simulink model "PID_Simulink_2DOF"  (R2019a)
settings: Solver=VariableStepAuto  StartTime=0.0  StopTime=250  RelTol=1e-3
undefined symbols (not defined in the file): A, A_d, B, B_d, C, C_d, DiscIntNeverNeededParam, Ki, Ki_d, Kx, Kx_d, Ts
libraries: simulink x6
settings Model: Creator=Caeta  LastModifiedBy=Caeta

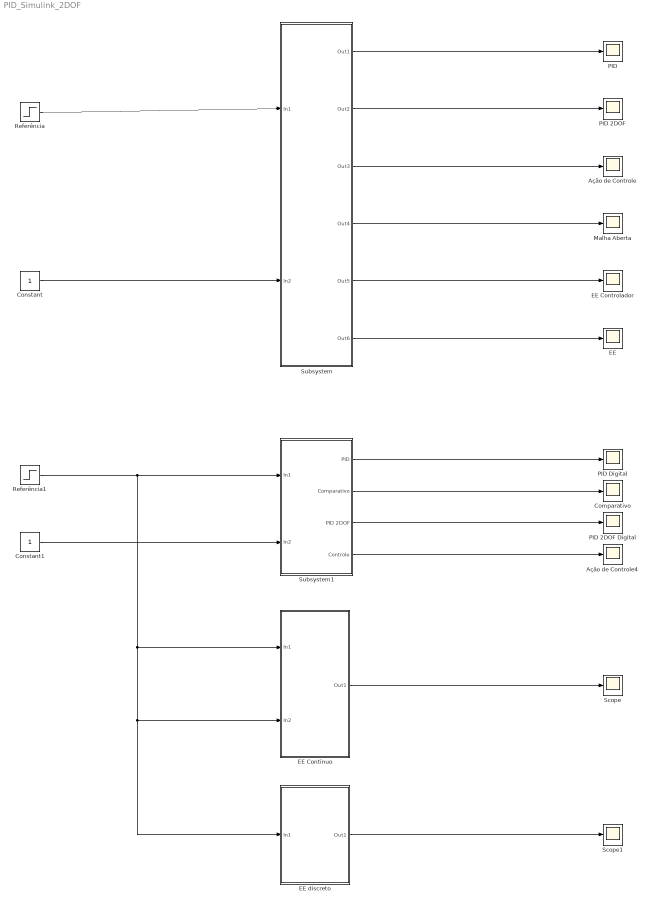
== system PID_Simulink_2DOF ==
  Ação de Controle : Scope
  Ação de Controle4 : Scope
  Comparativo : Scope
  Constant : Constant
  Constant1 : Constant
  "EE " : Scope
  EE Controlador : Scope
  EE Contínuo : Subsystem
  EE discreto : Subsystem
  Malha Aberta : Scope
  PID : Scope
  PID 2DOF : Scope
  PID 2DOF Digital : Scope
  PID Digital : Scope
  Referência : Step  Time=0  SampleTime=0
  Referência1 : Step  Time=0  SampleTime=Ts
  Scope : Scope
  Scope1 : Scope
  Subsystem : Subsystem
  Subsystem1 : Subsystem
  wires:
  Referência/1 -> Subsystem/1(In1)
  Constant/1 -> Subsystem/2(In2)
  Subsystem/1(Out1) -> PID/1
  Subsystem/2(Out2) -> PID 2DOF/1
  Subsystem/3(Out3) -> Ação de Controle/1
  Subsystem/4(Out4) -> Malha Aberta/1
  Subsystem/5(Out5) -> EE Controlador/1
  Subsystem/6(Out6) -> "EE "/1
  Constant1/1 -> Subsystem1/2(In2)
  Subsystem1/1(PID) -> PID Digital/1
  Subsystem1/2(Comparativo) -> Comparativo/1
  Subsystem1/3(PID 2DOF) -> PID 2DOF Digital/1
  Subsystem1/4(Controle) -> Ação de Controle4/1
  Referência1/1 -> EE Contínuo/1(In1), EE discreto/1(In1), EE Contínuo/2(In2), Subsystem1/1(In1)
  EE Contínuo/1(Out1) -> Scope/1
  EE discreto/1(Out1) -> Scope1/1

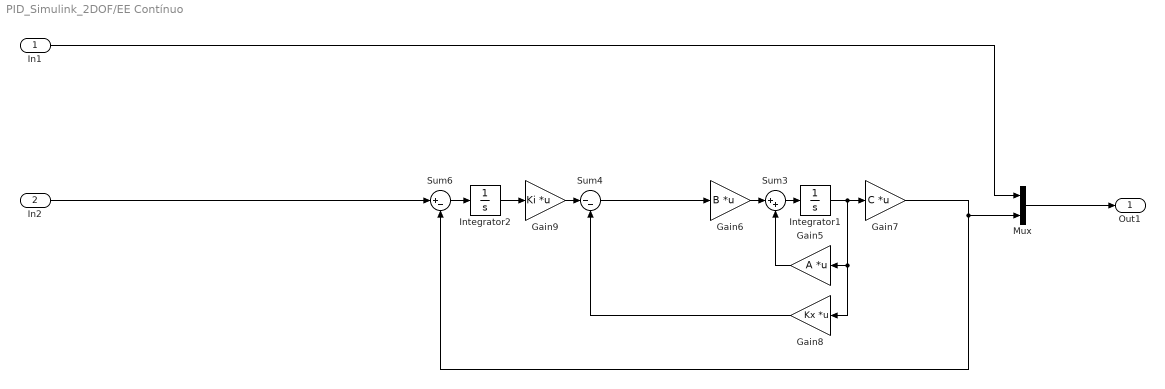
== system PID_Simulink_2DOF/EE Contínuo ==
  In1 : Inport
  In2 : Inport  Port=2
  Gain5 : Gain  Gain=A  Multiplication=Matrix(K*u)
  Gain6 : Gain  Gain=B  Multiplication=Matrix(K*u)
  Gain7 : Gain  Gain=C  Multiplication=Matrix(K*u)
  Gain8 : Gain  Gain=Kx  Multiplication=Matrix(K*u)
  Gain9 : Gain  Gain=Ki  Multiplication=Matrix(K*u)
  Integrator1 : Integrator
  Integrator2 : Integrator
  Mux : Mux  Inputs=2
  Sum3 : Sum  Inputs=|++
  Sum4 : Sum  Inputs=|--
  Sum6 : Sum  Inputs=|+-
  Out1 : Outport
  wires:
  Gain7/1 -> Mux/2, Sum6/2
  Gain9/1 -> Sum4/1
  Sum6/1 -> Integrator2/1
  Gain8/1 -> Sum4/2
  Integrator1/1 -> Gain8/1, Gain5/1, Gain7/1
  Gain6/1 -> Sum3/1
  Gain5/1 -> Sum3/2
  Sum3/1 -> Integrator1/1
  Integrator2/1 -> Gain9/1
  Sum4/1 -> Gain6/1
  In2/1 -> Sum6/1
  In1/1 -> Mux/1
  Mux/1 -> Out1/1

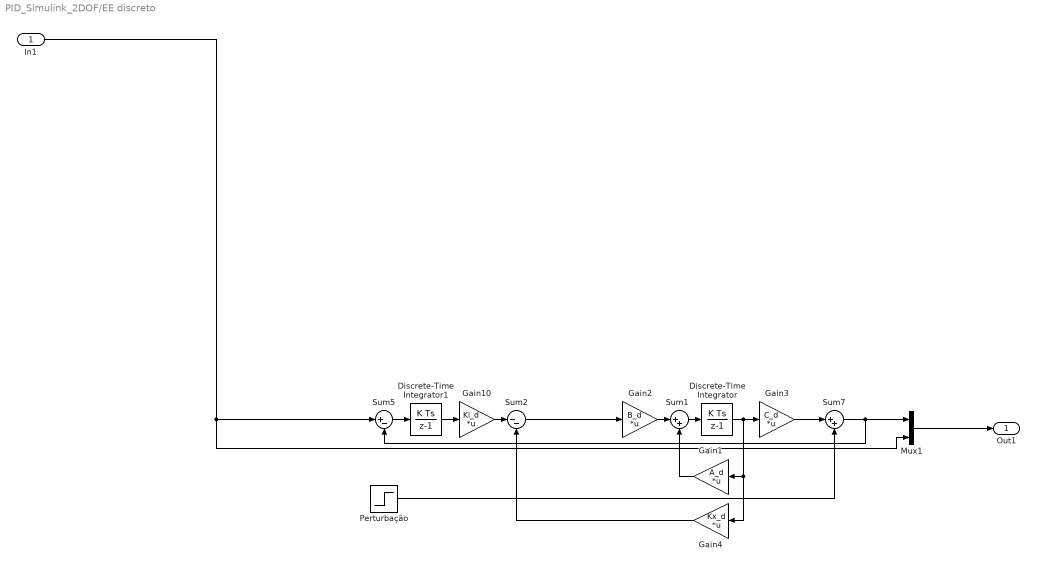
== system PID_Simulink_2DOF/EE discreto ==
  In1 : Inport
  Discrete-Time Integrator : DiscreteIntegrator  SampleTime=Ts  ICPrevOutput=DiscIntNeverNeededParam  ICPrevScaledInput=DiscIntNeverNeededParam
  Discrete-Time Integrator1 : DiscreteIntegrator  SampleTime=Ts  ICPrevOutput=DiscIntNeverNeededParam  ICPrevScaledInput=DiscIntNeverNeededParam
  Gain1 : Gain  Gain=A_d  Multiplication=Matrix(K*u)
  Gain10 : Gain  Gain=Ki_d  Multiplication=Matrix(K*u)
  Gain2 : Gain  Gain=B_d  Multiplication=Matrix(K*u)
  Gain3 : Gain  Gain=C_d  Multiplication=Matrix(K*u)
  Gain4 : Gain  Gain=Kx_d  Multiplication=Matrix(K*u)
  Mux1 : Mux  Inputs=2
  Perturbação : Step  Time=150  After=0.1  SampleTime=Ts
  Sum1 : Sum  Inputs=|++
  Sum2 : Sum  Inputs=|--
  Sum5 : Sum  Inputs=|+-
  Sum7 : Sum  Inputs=|++
  Out1 : Outport
  wires:
  Sum7/1 -> Mux1/1, Sum5/2
  Perturbação/1 -> Sum7/2
  Gain2/1 -> Sum1/1
  Gain10/1 -> Sum2/1
  Discrete-Time Integrator/1 -> Gain4/1, Gain1/1, Gain3/1
  Discrete-Time Integrator1/1 -> Gain10/1
  Mux1/1 -> Out1/1
  Gain4/1 -> Sum2/2
  Sum1/1 -> Discrete-Time Integrator/1
  In1/1 -> Mux1/2, Sum5/1
  Sum5/1 -> Discrete-Time Integrator1/1
  Gain1/1 -> Sum1/2
  Sum2/1 -> Gain2/1
  Gain3/1 -> Sum7/1

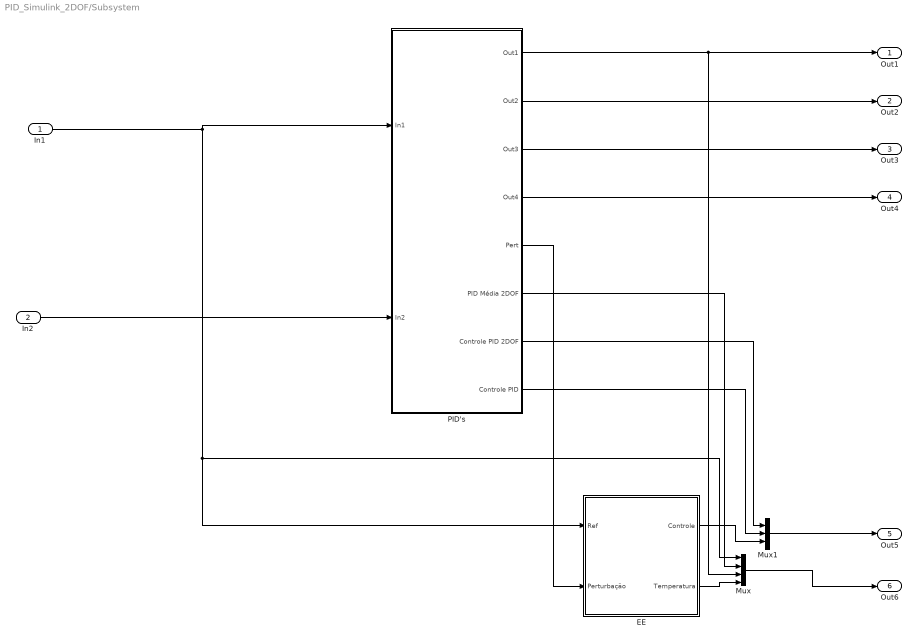
== system PID_Simulink_2DOF/Subsystem ==
  In1 : Inport
  In2 : Inport  Port=2
  EE : Subsystem
  Mux : Mux
  Mux1 : Mux  Inputs=3
  PID's : Subsystem
  Out1 : Outport
  Out2 : Outport  Port=2
  Out3 : Outport  Port=3
  Out4 : Outport  Port=4
  Out5 : Outport  Port=5
  Out6 : Outport  Port=6
  wires:
  PID's/3(Out3) -> Out3/1
  PID's/8(Controle PID) -> Mux1/2
  Mux1/1 -> Out5/1
  PID's/6(PID Média 2DOF) -> Mux/2
  In1/1 -> Mux/1, EE/1(Ref), PID's/1(In1)
  PID's/5(Pert) -> EE/2(Perturbação)
  PID's/7(Controle PID 2DOF) -> Mux1/1
  PID's/1(Out1) -> Out1/1, Mux/3
  PID's/4(Out4) -> Out4/1
  PID's/2(Out2) -> Out2/1
  In2/1 -> PID's/2(In2)
  Mux/1 -> Out6/1
  EE/1(Controle) -> Mux1/3
  EE/2(Temperatura) -> Mux/4

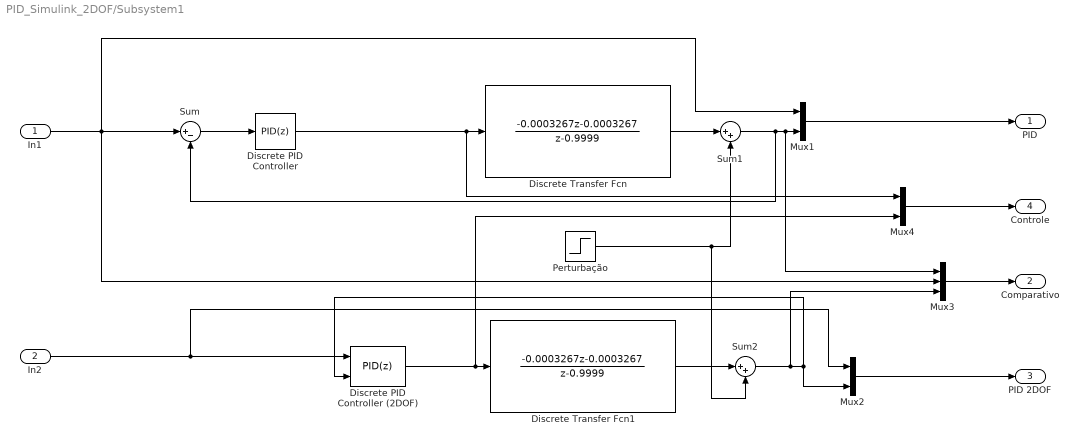
== system PID_Simulink_2DOF/Subsystem1 ==
  In1 : Inport
  In2 : Inport  Port=2
  Discrete Transfer Fcn : DiscreteTransferFcn  Numerator=[-0.0003267 -0.0003267]  Denominator=[1 -0.9999]  SampleTime=Ts
  Discrete Transfer Fcn1 : DiscreteTransferFcn  Numerator=[-0.0003267 -0.0003267]  Denominator=[1 -0.9999]  SampleTime=Ts
  Discrete PID Controller : simulink/Continuous/PID Controller  Controller=PID  Form=Parallel  TimeDomain=Discrete-time  SampleTime=Ts  IntegratorMethod=Forward Euler  FilterMethod=Forward Euler  ControllerParametersSource=internal  P=-38  I=-3  D=-0.1  UseFilter=off  N=0  TunerSelectOption=Transfer Function Based (PID Tuner App)  InitialConditionSource=internal  InitialConditionForIntegrator=0  InitialConditionForFilter=0  DifferentiatorICPrevScaledInput=0  ExternalReset=none  TrackingMode=off  Kt=1  LimitOutput=off  UpperSaturationLimit=inf  LowerSaturationLimit=-inf  LinearizeAsGain=off  AntiWindupMode=none  Kb=1  POutMin=[]  POutMax=[]  IOutMin=[]  IOutMax=[]  DOutMin=[]  DOutMax=[]  NOutMin=[]  NOutMax=[]  SumOutMin=[]  SumOutMax=[]  SaturationOutMin=[]  SaturationOutMax=[]  PParamMin=[]  PParamMax=[]  IParamMin=[]  IParamMax=[]  DParamMin=[]  DParamMax=[]  NParamMin=[]  NParamMax=[]  KbParamMin=[]  KbParamMax=[]  KtParamMin=[]  KtParamMax=[]  KbOutMin=[]  KbOutMax=[]  KtOutMin=[]  KtOutMax=[]  IntegratorOutMin=[]  IntegratorOutMax=[]  FilterOutMin=[]  FilterOutMax=[]  SumI1OutMin=[]  SumI1OutMax=[]  SumI2OutMin=[]  SumI2OutMax=[]  SumI3OutMin=[]  SumI3OutMax=[]  SumI4OutMin=[]  SumI4OutMax=[]  SumDOutMin=[]  SumDOutMax=[]  DifferentiatorOutMin=[]  DifferentiatorOutMax=[]  FilterDiffOutCoefMin=[]  FilterDiffOutCoefMax=[]  ReciprocalOutMin=[]  ReciprocalOutMax=[]  SumDenOutMin=[]  SumDenOutMax=[]  SumNumOutMin=[]  SumNumOutMax=[]  DivideOutMin=[]  DivideOutMax=[]  IntegratorContinuousStateAttributes=''  IntegratorStateMustResolveToSignalObject=off  IntegratorRTWStateStorageClass=Auto  FilterContinuousStateAttributes=''  FilterStateMustResolveToSignalObject=off  FilterRTWStateStorageClass=Auto  ParallelPVariant=InternalParameters  IdealPVariant=Disabled  IVariant=InternalParameters  DVariant=InternalParameters  IntegratorVariant=Discrete  SatVariant=Disabled  AWVariant=Passthrough  PCopyVariant=Disabled  TRVariant=Disabled  FdbkBlocksVariant=Forward  IdealPFdbkVariant=Disabled  SatFdbkVariant=Disabled  DerivativeFilterVariant=Differentiator  NVariant=Passthrough  NCopyVariant=Disabled_SignalSpec  FilterICVariant=InternalICsDifferentiator  IntegratorICVariant=InternalICs  ExternalResetVariant=Disabled  TRSumVariant=Passthrough  SumFdbkVariant=Disabled  SumVariant=Sum_PID
  Discrete PID Controller (2DOF) : simulink/Continuous/PID Controller (2DOF)  Controller=PID  Form=Parallel  TimeDomain=Discrete-time  SampleTime=Ts  IntegratorMethod=Forward Euler  FilterMethod=Forward Euler  ControllerParametersSource=internal  P=-38  I=-3  D=-0.1  UseFilter=on  N=0  b=0.8  c=0.8  TunerSelectOption=Transfer Function Based (PID Tuner App)  InitialConditionSource=internal  InitialConditionForIntegrator=0  InitialConditionForFilter=0  DifferentiatorICPrevScaledInput=0  ExternalReset=none  TrackingMode=off  Kt=1  LimitOutput=off  UpperSaturationLimit=inf  LowerSaturationLimit=-inf  LinearizeAsGain=off  AntiWindupMode=none  Kb=1  POutMin=[]  POutMax=[]  IOutMin=[]  IOutMax=[]  DOutMin=[]  DOutMax=[]  NOutMin=[]  NOutMax=[]  bOutMin=[]  bOutMax=[]  cOutMin=[]  cOutMax=[]  SumOutMin=[]  SumOutMax=[]  SaturationOutMin=[]  SaturationOutMax=[]  PParamMin=[]  PParamMax=[]  IParamMin=[]  IParamMax=[]  DParamMin=[]  DParamMax=[]  NParamMin=[]  NParamMax=[]  bParamMin=[]  bParamMax=[]  cParamMin=[]  cParamMax=[]  KbParamMin=[]  KbParamMax=[]  KtParamMin=[]  KtParamMax=[]  KbOutMin=[]  KbOutMax=[]  KtOutMin=[]  KtOutMax=[]  IntegratorOutMin=[]  IntegratorOutMax=[]  FilterOutMin=[]  FilterOutMax=[]  SumI1OutMin=[]  SumI1OutMax=[]  SumI2OutMin=[]  SumI2OutMax=[]  SumI3OutMin=[]  SumI3OutMax=[]  SumI4OutMin=[]  SumI4OutMax=[]  SumDOutMin=[]  SumDOutMax=[]  Sum1OutMin=[]  Sum1OutMax=[]  Sum2OutMin=[]  Sum2OutMax=[]  Sum3OutMin=[]  Sum3OutMax=[]  DifferentiatorOutMin=[]  DifferentiatorOutMax=[]  FilterDiffOutCoefMin=[]  FilterDiffOutCoefMax=[]  ReciprocalOutMin=[]  ReciprocalOutMax=[]  SumDenOutMin=[]  SumDenOutMax=[]  SumNumOutMin=[]  SumNumOutMax=[]  DivideOutMin=[]  DivideOutMax=[]  IntegratorContinuousStateAttributes=''  IntegratorStateMustResolveToSignalObject=off  IntegratorRTWStateStorageClass=Auto  FilterContinuousStateAttributes=''  FilterStateMustResolveToSignalObject=off  FilterRTWStateStorageClass=Auto  ParallelPVariant=InternalParameters  IdealPVariant=Disabled  IVariant=InternalParameters  DVariant=InternalParameters  bVariant=InternalParameters  cVariant=InternalParameters  IntegratorVariant=Discrete  SatVariant=Disabled  AWVariant=Passthrough  PCopyVariant=Disabled  TRVariant=Disabled  FdbkBlocksVariant=Forward  IdealPFdbkVariant=Disabled  SatFdbkVariant=Disabled  DerivativeFilterVariant=ForwardEulerFilter  NVariant=InternalParameters  NCopyVariant=Disabled  FilterICVariant=InternalICsFilter  IntegratorICVariant=InternalICs  ExternalResetVariant=Disabled  TRSumVariant=Passthrough  SumFdbkVariant=Disabled  SumVariant=Sum_PID
  Mux1 : Mux  Inputs=2
  Mux2 : Mux  Inputs=2
  Mux3 : Mux  Inputs=3
  Mux4 : Mux  Inputs=2
  Perturbação : Step  Time=50  After=0.1  SampleTime=Ts
  Sum : Sum  Inputs=|+-
  Sum1 : Sum  Inputs=|++
  Sum2 : Sum  Inputs=|++
  PID : Outport
  Comparativo : Outport  Port=2
  PID 2DOF : Outport  Port=3
  Controle : Outport  Port=4
  wires:
  Sum2/1 -> Mux3/3, Mux2/2, Discrete PID Controller (2DOF)/2
  Discrete Transfer Fcn/1 -> Sum1/1
  In1/1 -> Mux3/2, Mux1/1, Sum/1
  Sum/1 -> Discrete PID Controller/1
  In2/1 -> Mux2/1, Discrete PID Controller (2DOF)/1
  Perturbação/1 -> Sum2/2, Sum1/2
  Sum1/1 -> Sum/2, Mux3/1, Mux1/2
  Discrete Transfer Fcn1/1 -> Sum2/1
  Mux3/1 -> Comparativo/1
  Mux1/1 -> PID/1
  Mux2/1 -> PID 2DOF/1
  Discrete PID Controller (2DOF)/1 -> Mux4/2, Discrete Transfer Fcn1/1
  Discrete PID Controller/1 -> Mux4/1, Discrete Transfer Fcn/1
  Mux4/1 -> Controle/1

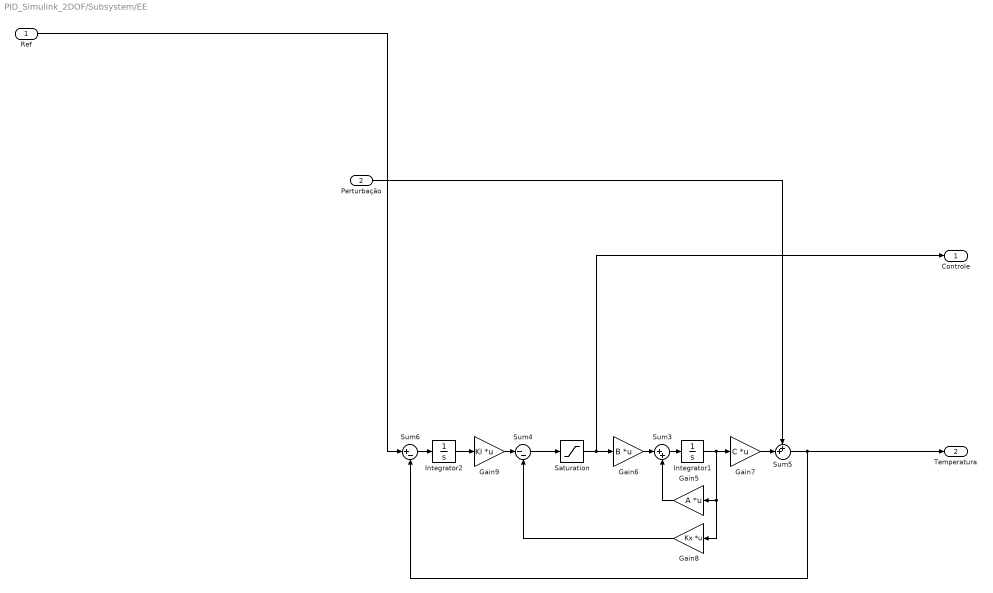
== system PID_Simulink_2DOF/Subsystem/EE ==
  Ref : Inport
  Perturbação : Inport  Port=2
  Gain5 : Gain  Gain=A  Multiplication=Matrix(K*u)
  Gain6 : Gain  Gain=B  Multiplication=Matrix(K*u)
  Gain7 : Gain  Gain=C  Multiplication=Matrix(K*u)
  Gain8 : Gain  Gain=Kx  Multiplication=Matrix(K*u)
  Gain9 : Gain  Gain=Ki  Multiplication=Matrix(K*u)
  Integrator1 : Integrator
  Integrator2 : Integrator
  Saturation : Saturate  UpperLimit=255  LowerLimit=0
  Sum3 : Sum  Inputs=|++
  Sum4 : Sum  Inputs=|--
  Sum5 : Sum  Inputs=++|
  Sum6 : Sum  Inputs=|+-
  Controle : Outport
  Temperatura : Outport  Port=2
  wires:
  Sum3/1 -> Integrator1/1
  Sum5/1 -> Sum6/2, Temperatura/1
  Gain9/1 -> Sum4/1
  Integrator2/1 -> Gain9/1
  Sum6/1 -> Integrator2/1
  Gain6/1 -> Sum3/1
  Gain7/1 -> Sum5/2
  Gain8/1 -> Sum4/2
  Integrator1/1 -> Gain8/1, Gain5/1, Gain7/1
  Gain5/1 -> Sum3/2
  Perturbação/1 -> Sum5/1
  Ref/1 -> Sum6/1
  Sum4/1 -> Saturation/1
  Saturation/1 -> Controle/1, Gain6/1

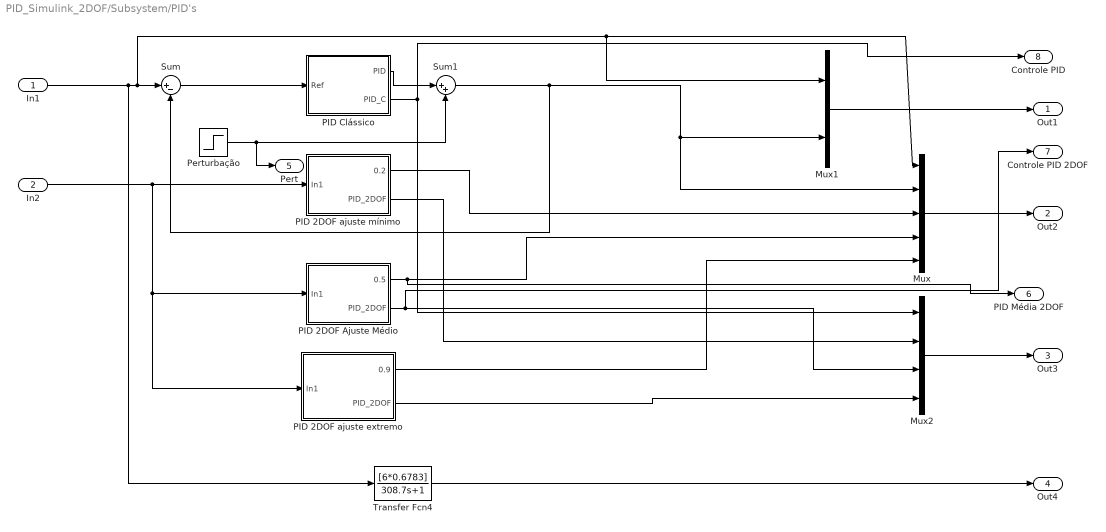
== system PID_Simulink_2DOF/Subsystem/PID's ==
  In1 : Inport
  In2 : Inport  Port=2
  Mux : Mux  Inputs=5
  Mux1 : Mux  Inputs=2
  Mux2 : Mux
  PID 2DOF Ajuste Médio : Subsystem
  PID 2DOF ajuste extremo : Subsystem
  PID 2DOF ajuste mínimo : Subsystem
  PID Clássico : Subsystem
  Perturbação : Step  Time=150  After=0.1  SampleTime=0
  Sum : Sum  Inputs=|+-
  Sum1 : Sum  Inputs=|++
  Transfer Fcn4 : TransferFcn  Numerator=[6*0.6783]  Denominator=[308.7 1]
  Out1 : Outport
  Out2 : Outport  Port=2
  Out3 : Outport  Port=3
  Out4 : Outport  Port=4
  Pert : Outport  Port=5
  PID Média 2DOF : Outport  Port=6
  Controle PID 2DOF : Outport  Port=7
  Controle PID : Outport  Port=8
  wires:
  Sum/1 -> PID Clássico/1(Ref)
  In2/1 -> PID 2DOF Ajuste Médio/1(In1), PID 2DOF ajuste extremo/1(In1), PID 2DOF ajuste mínimo/1(In1)
  Sum1/1 -> Mux1/2, Mux/2, Sum/2
  Mux/1 -> Out2/1
  PID 2DOF Ajuste Médio/2(PID_2DOF) -> Controle PID 2DOF/1, Mux2/3
  In1/1 -> Transfer Fcn4/1, Mux1/1, Mux/1, Sum/1
  PID 2DOF ajuste mínimo/1(0.2) -> Mux/3
  Transfer Fcn4/1 -> Out4/1
  PID Clássico/1(PID) -> Sum1/1
  PID 2DOF Ajuste Médio/1(0.5) -> PID Média 2DOF/1, Mux/4
  PID 2DOF ajuste mínimo/2("PID_2DOF ") -> Mux2/2
  PID 2DOF ajuste extremo/2(PID_2DOF) -> Mux2/4
  PID Clássico/2(PID_C) -> Mux2/1, Controle PID/1
  PID 2DOF ajuste extremo/1("0.9 ") -> Mux/5
  Perturbação/1 -> Pert/1, Sum1/2
  Mux1/1 -> Out1/1
  Mux2/1 -> Out3/1

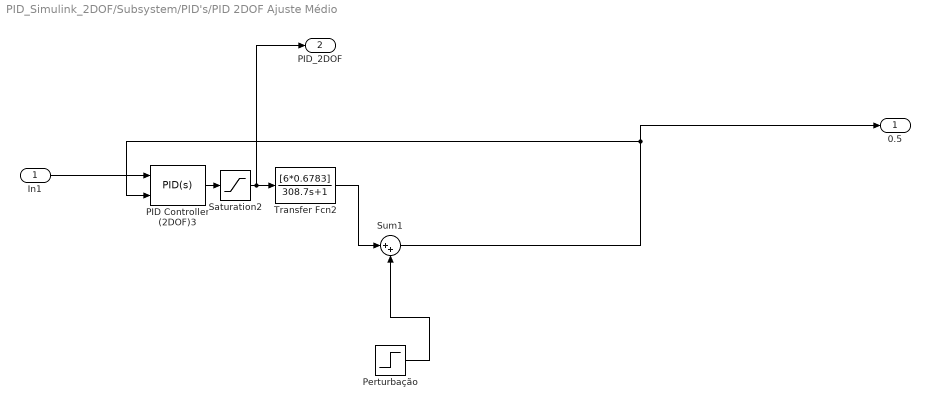
== system PID_Simulink_2DOF/Subsystem/PID's/PID 2DOF Ajuste Médio ==
  In1 : Inport
  PID Controller (2DOF)3 : simulink/Continuous/PID Controller (2DOF)  Controller=PID  Form=Parallel  TimeDomain=Continuous-time  SampleTime=-1  IntegratorMethod=Forward Euler  FilterMethod=Forward Euler  ControllerParametersSource=internal  P=7.03  I=0.182  D=25.1  UseFilter=on  N=0  b=0.5  c=0.5  TunerSelectOption=Transfer Function Based (PID Tuner App)  InitialConditionSource=internal  InitialConditionForIntegrator=0  InitialConditionForFilter=0  DifferentiatorICPrevScaledInput=0  ExternalReset=none  TrackingMode=off  Kt=1  LimitOutput=off  UpperSaturationLimit=inf  LowerSaturationLimit=-inf  LinearizeAsGain=on  AntiWindupMode=none  Kb=1  POutMin=[]  POutMax=[]  IOutMin=[]  IOutMax=[]  DOutMin=[]  DOutMax=[]  NOutMin=[]  NOutMax=[]  bOutMin=[]  bOutMax=[]  cOutMin=[]  cOutMax=[]  SumOutMin=[]  SumOutMax=[]  SaturationOutMin=[]  SaturationOutMax=[]  PParamMin=[]  PParamMax=[]  IParamMin=[]  IParamMax=[]  DParamMin=[]  DParamMax=[]  NParamMin=[]  NParamMax=[]  bParamMin=[]  bParamMax=[]  cParamMin=[]  cParamMax=[]  KbParamMin=[]  KbParamMax=[]  KtParamMin=[]  KtParamMax=[]  KbOutMin=[]  KbOutMax=[]  KtOutMin=[]  KtOutMax=[]  IntegratorOutMin=[]  IntegratorOutMax=[]  FilterOutMin=[]  FilterOutMax=[]  SumI1OutMin=[]  SumI1OutMax=[]  SumI2OutMin=[]  SumI2OutMax=[]  SumI3OutMin=[]  SumI3OutMax=[]  SumI4OutMin=[]  SumI4OutMax=[]  SumDOutMin=[]  SumDOutMax=[]  Sum1OutMin=[]  Sum1OutMax=[]  Sum2OutMin=[]  Sum2OutMax=[]  Sum3OutMin=[]  Sum3OutMax=[]  DifferentiatorOutMin=[]  DifferentiatorOutMax=[]  FilterDiffOutCoefMin=[]  FilterDiffOutCoefMax=[]  ReciprocalOutMin=[]  ReciprocalOutMax=[]  SumDenOutMin=[]  SumDenOutMax=[]  SumNumOutMin=[]  SumNumOutMax=[]  DivideOutMin=[]  DivideOutMax=[]  IntegratorContinuousStateAttributes=''  IntegratorStateMustResolveToSignalObject=off  IntegratorRTWStateStorageClass=Auto  FilterContinuousStateAttributes=''  FilterStateMustResolveToSignalObject=off  FilterRTWStateStorageClass=Auto  ParallelPVariant=InternalParameters  IdealPVariant=Disabled  IVariant=InternalParameters  DVariant=InternalParameters  bVariant=InternalParameters  cVariant=InternalParameters  IntegratorVariant=Continuous  SatVariant=Disabled  AWVariant=Passthrough  PCopyVariant=Disabled  TRVariant=Disabled  FdbkBlocksVariant=Forward  IdealPFdbkVariant=Disabled  SatFdbkVariant=Disabled  DerivativeFilterVariant=ContFilter  NVariant=InternalParameters  NCopyVariant=Disabled  FilterICVariant=InternalICsFilter  IntegratorICVariant=InternalICs  ExternalResetVariant=Disabled  TRSumVariant=Passthrough  SumFdbkVariant=Disabled  SumVariant=Sum_PID
  Perturbação : Step  Time=150  After=0.1  SampleTime=0
  Saturation2 : Saturate  UpperLimit=255  LowerLimit=0
  Sum1 : Sum  Inputs=|++
  Transfer Fcn2 : TransferFcn  Numerator=[6*0.6783]  Denominator=[308.7 1]
  0.5 : Outport
  PID_2DOF : Outport  Port=2
  wires:
  PID Controller (2DOF)3/1 -> Saturation2/1
  In1/1 -> PID Controller (2DOF)3/1
  Saturation2/1 -> PID_2DOF/1, Transfer Fcn2/1
  Perturbação/1 -> Sum1/2
  Transfer Fcn2/1 -> Sum1/1
  Sum1/1 -> 0.5/1, PID Controller (2DOF)3/2

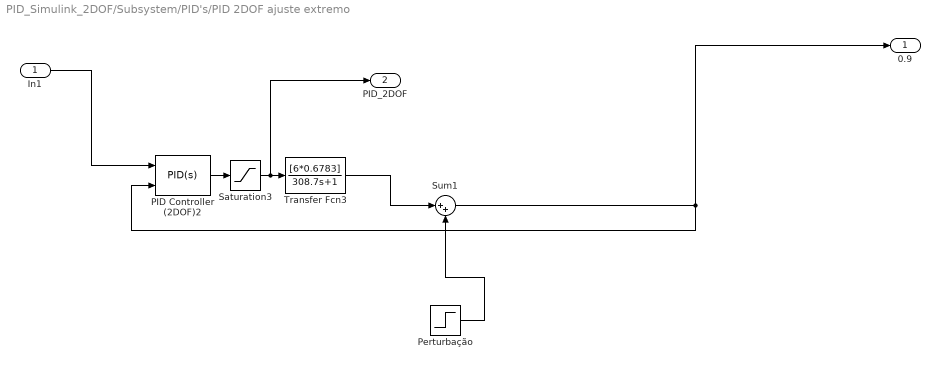
== system PID_Simulink_2DOF/Subsystem/PID's/PID 2DOF ajuste extremo ==
  In1 : Inport
  PID Controller (2DOF)2 : simulink/Continuous/PID Controller (2DOF)  Controller=PID  Form=Parallel  TimeDomain=Continuous-time  SampleTime=-1  IntegratorMethod=Forward Euler  FilterMethod=Forward Euler  ControllerParametersSource=internal  P=7.03  I=0.182  D=25.1  UseFilter=on  N=0  b=0.9  c=0.9  TunerSelectOption=Transfer Function Based (PID Tuner App)  InitialConditionSource=internal  InitialConditionForIntegrator=0  InitialConditionForFilter=0  DifferentiatorICPrevScaledInput=0  ExternalReset=none  TrackingMode=off  Kt=1  LimitOutput=off  UpperSaturationLimit=inf  LowerSaturationLimit=-inf  LinearizeAsGain=on  AntiWindupMode=none  Kb=1  POutMin=[]  POutMax=[]  IOutMin=[]  IOutMax=[]  DOutMin=[]  DOutMax=[]  NOutMin=[]  NOutMax=[]  bOutMin=[]  bOutMax=[]  cOutMin=[]  cOutMax=[]  SumOutMin=[]  SumOutMax=[]  SaturationOutMin=[]  SaturationOutMax=[]  PParamMin=[]  PParamMax=[]  IParamMin=[]  IParamMax=[]  DParamMin=[]  DParamMax=[]  NParamMin=[]  NParamMax=[]  bParamMin=[]  bParamMax=[]  cParamMin=[]  cParamMax=[]  KbParamMin=[]  KbParamMax=[]  KtParamMin=[]  KtParamMax=[]  KbOutMin=[]  KbOutMax=[]  KtOutMin=[]  KtOutMax=[]  IntegratorOutMin=[]  IntegratorOutMax=[]  FilterOutMin=[]  FilterOutMax=[]  SumI1OutMin=[]  SumI1OutMax=[]  SumI2OutMin=[]  SumI2OutMax=[]  SumI3OutMin=[]  SumI3OutMax=[]  SumI4OutMin=[]  SumI4OutMax=[]  SumDOutMin=[]  SumDOutMax=[]  Sum1OutMin=[]  Sum1OutMax=[]  Sum2OutMin=[]  Sum2OutMax=[]  Sum3OutMin=[]  Sum3OutMax=[]  DifferentiatorOutMin=[]  DifferentiatorOutMax=[]  FilterDiffOutCoefMin=[]  FilterDiffOutCoefMax=[]  ReciprocalOutMin=[]  ReciprocalOutMax=[]  SumDenOutMin=[]  SumDenOutMax=[]  SumNumOutMin=[]  SumNumOutMax=[]  DivideOutMin=[]  DivideOutMax=[]  IntegratorContinuousStateAttributes=''  IntegratorStateMustResolveToSignalObject=off  IntegratorRTWStateStorageClass=Auto  FilterContinuousStateAttributes=''  FilterStateMustResolveToSignalObject=off  FilterRTWStateStorageClass=Auto  ParallelPVariant=InternalParameters  IdealPVariant=Disabled  IVariant=InternalParameters  DVariant=InternalParameters  bVariant=InternalParameters  cVariant=InternalParameters  IntegratorVariant=Continuous  SatVariant=Disabled  AWVariant=Passthrough  PCopyVariant=Disabled  TRVariant=Disabled  FdbkBlocksVariant=Forward  IdealPFdbkVariant=Disabled  SatFdbkVariant=Disabled  DerivativeFilterVariant=ContFilter  NVariant=InternalParameters  NCopyVariant=Disabled  FilterICVariant=InternalICsFilter  IntegratorICVariant=InternalICs  ExternalResetVariant=Disabled  TRSumVariant=Passthrough  SumFdbkVariant=Disabled  SumVariant=Sum_PID
  Perturbação : Step  Time=150  After=0.1  SampleTime=0
  Saturation3 : Saturate  UpperLimit=255  LowerLimit=0
  Sum1 : Sum  Inputs=|++
  Transfer Fcn3 : TransferFcn  Numerator=[6*0.6783]  Denominator=[308.7 1]
  "0.9 " : Outport
  PID_2DOF : Outport  Port=2
  wires:
  Saturation3/1 -> PID_2DOF/1, Transfer Fcn3/1
  PID Controller (2DOF)2/1 -> Saturation3/1
  In1/1 -> PID Controller (2DOF)2/1
  Sum1/1 -> PID Controller (2DOF)2/2, "0.9 "/1
  Perturbação/1 -> Sum1/2
  Transfer Fcn3/1 -> Sum1/1

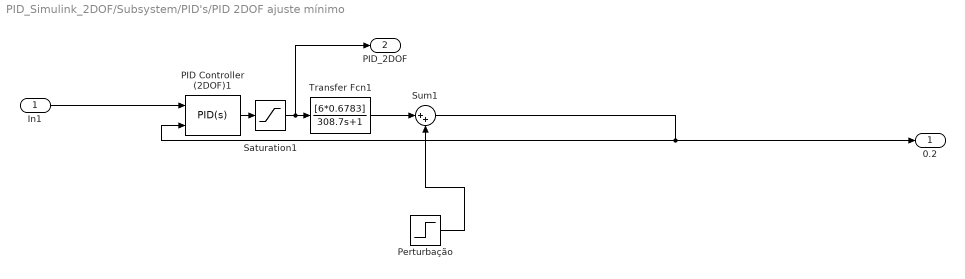
== system PID_Simulink_2DOF/Subsystem/PID's/PID 2DOF ajuste mínimo ==
  In1 : Inport
  PID Controller (2DOF)1 : simulink/Continuous/PID Controller (2DOF)  Controller=PID  Form=Parallel  TimeDomain=Continuous-time  SampleTime=-1  IntegratorMethod=Forward Euler  FilterMethod=Forward Euler  ControllerParametersSource=internal  P=7.03  I=0.182  D=25.1  UseFilter=on  N=0  b=0.2  c=0.2  TunerSelectOption=Transfer Function Based (PID Tuner App)  InitialConditionSource=internal  InitialConditionForIntegrator=0  InitialConditionForFilter=0  DifferentiatorICPrevScaledInput=0  ExternalReset=none  TrackingMode=off  Kt=1  LimitOutput=off  UpperSaturationLimit=inf  LowerSaturationLimit=-inf  LinearizeAsGain=on  AntiWindupMode=none  Kb=1  POutMin=[]  POutMax=[]  IOutMin=[]  IOutMax=[]  DOutMin=[]  DOutMax=[]  NOutMin=[]  NOutMax=[]  bOutMin=[]  bOutMax=[]  cOutMin=[]  cOutMax=[]  SumOutMin=[]  SumOutMax=[]  SaturationOutMin=[]  SaturationOutMax=[]  PParamMin=[]  PParamMax=[]  IParamMin=[]  IParamMax=[]  DParamMin=[]  DParamMax=[]  NParamMin=[]  NParamMax=[]  bParamMin=[]  bParamMax=[]  cParamMin=[]  cParamMax=[]  KbParamMin=[]  KbParamMax=[]  KtParamMin=[]  KtParamMax=[]  KbOutMin=[]  KbOutMax=[]  KtOutMin=[]  KtOutMax=[]  IntegratorOutMin=[]  IntegratorOutMax=[]  FilterOutMin=[]  FilterOutMax=[]  SumI1OutMin=[]  SumI1OutMax=[]  SumI2OutMin=[]  SumI2OutMax=[]  SumI3OutMin=[]  SumI3OutMax=[]  SumI4OutMin=[]  SumI4OutMax=[]  SumDOutMin=[]  SumDOutMax=[]  Sum1OutMin=[]  Sum1OutMax=[]  Sum2OutMin=[]  Sum2OutMax=[]  Sum3OutMin=[]  Sum3OutMax=[]  DifferentiatorOutMin=[]  DifferentiatorOutMax=[]  FilterDiffOutCoefMin=[]  FilterDiffOutCoefMax=[]  ReciprocalOutMin=[]  ReciprocalOutMax=[]  SumDenOutMin=[]  SumDenOutMax=[]  SumNumOutMin=[]  SumNumOutMax=[]  DivideOutMin=[]  DivideOutMax=[]  IntegratorContinuousStateAttributes=''  IntegratorStateMustResolveToSignalObject=off  IntegratorRTWStateStorageClass=Auto  FilterContinuousStateAttributes=''  FilterStateMustResolveToSignalObject=off  FilterRTWStateStorageClass=Auto  ParallelPVariant=InternalParameters  IdealPVariant=Disabled  IVariant=InternalParameters  DVariant=InternalParameters  bVariant=InternalParameters  cVariant=InternalParameters  IntegratorVariant=Continuous  SatVariant=Disabled  AWVariant=Passthrough  PCopyVariant=Disabled  TRVariant=Disabled  FdbkBlocksVariant=Forward  IdealPFdbkVariant=Disabled  SatFdbkVariant=Disabled  DerivativeFilterVariant=ContFilter  NVariant=InternalParameters  NCopyVariant=Disabled  FilterICVariant=InternalICsFilter  IntegratorICVariant=InternalICs  ExternalResetVariant=Disabled  TRSumVariant=Passthrough  SumFdbkVariant=Disabled  SumVariant=Sum_PID
  Perturbação : Step  Time=150  After=0.1  SampleTime=0
  Saturation1 : Saturate  UpperLimit=255  LowerLimit=0
  Sum1 : Sum  Inputs=|++
  Transfer Fcn1 : TransferFcn  Numerator=[6*0.6783]  Denominator=[308.7 1]
  0.2 : Outport
  "PID_2DOF " : Outport  Port=2
  wires:
  PID Controller (2DOF)1/1 -> Saturation1/1
  Saturation1/1 -> "PID_2DOF "/1, Transfer Fcn1/1
  In1/1 -> PID Controller (2DOF)1/1
  Transfer Fcn1/1 -> Sum1/1
  Perturbação/1 -> Sum1/2
  Sum1/1 -> PID Controller (2DOF)1/2, 0.2/1

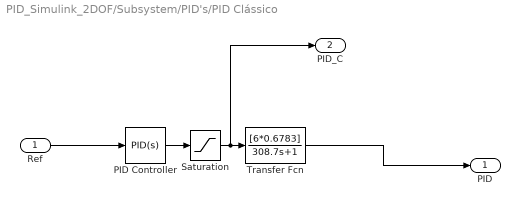
== system PID_Simulink_2DOF/Subsystem/PID's/PID Clássico ==
  Ref : Inport
  PID Controller : simulink/Continuous/PID Controller  Controller=PID  Form=Parallel  TimeDomain=Continuous-time  SampleTime=-1  IntegratorMethod=Forward Euler  FilterMethod=Forward Euler  ControllerParametersSource=internal  P=7.03  I=0.182  D=25.1  UseFilter=on  N=0  TunerSelectOption=Transfer Function Based (PID Tuner App)  InitialConditionSource=internal  InitialConditionForIntegrator=0  InitialConditionForFilter=0  DifferentiatorICPrevScaledInput=0  ExternalReset=none  TrackingMode=off  Kt=1  LimitOutput=off  UpperSaturationLimit=inf  LowerSaturationLimit=-inf  LinearizeAsGain=on  AntiWindupMode=none  Kb=1  POutMin=[]  POutMax=[]  IOutMin=[]  IOutMax=[]  DOutMin=[]  DOutMax=[]  NOutMin=[]  NOutMax=[]  SumOutMin=[]  SumOutMax=[]  SaturationOutMin=[]  SaturationOutMax=[]  PParamMin=[]  PParamMax=[]  IParamMin=[]  IParamMax=[]  DParamMin=[]  DParamMax=[]  NParamMin=[]  NParamMax=[]  KbParamMin=[]  KbParamMax=[]  KtParamMin=[]  KtParamMax=[]  KbOutMin=[]  KbOutMax=[]  KtOutMin=[]  KtOutMax=[]  IntegratorOutMin=[]  IntegratorOutMax=[]  FilterOutMin=[]  FilterOutMax=[]  SumI1OutMin=[]  SumI1OutMax=[]  SumI2OutMin=[]  SumI2OutMax=[]  SumI3OutMin=[]  SumI3OutMax=[]  SumI4OutMin=[]  SumI4OutMax=[]  SumDOutMin=[]  SumDOutMax=[]  DifferentiatorOutMin=[]  DifferentiatorOutMax=[]  FilterDiffOutCoefMin=[]  FilterDiffOutCoefMax=[]  ReciprocalOutMin=[]  ReciprocalOutMax=[]  SumDenOutMin=[]  SumDenOutMax=[]  SumNumOutMin=[]  SumNumOutMax=[]  DivideOutMin=[]  DivideOutMax=[]  IntegratorContinuousStateAttributes=''  IntegratorStateMustResolveToSignalObject=off  IntegratorRTWStateStorageClass=Auto  FilterContinuousStateAttributes=''  FilterStateMustResolveToSignalObject=off  FilterRTWStateStorageClass=Auto  ParallelPVariant=InternalParameters  IdealPVariant=Disabled  IVariant=InternalParameters  DVariant=InternalParameters  IntegratorVariant=Continuous  SatVariant=Disabled  AWVariant=Passthrough  PCopyVariant=Disabled  TRVariant=Disabled  FdbkBlocksVariant=Forward  IdealPFdbkVariant=Disabled  SatFdbkVariant=Disabled  DerivativeFilterVariant=ContFilter  NVariant=InternalParameters  NCopyVariant=Disabled  FilterICVariant=InternalICsFilter  IntegratorICVariant=InternalICs  ExternalResetVariant=Disabled  TRSumVariant=Passthrough  SumFdbkVariant=Disabled  SumVariant=Sum_PID
  Saturation : Saturate  UpperLimit=255  LowerLimit=0
  Transfer Fcn : TransferFcn  Numerator=[6*0.6783]  Denominator=[308.7 1]
  PID : Outport
  PID_C : Outport  Port=2
  wires:
  Saturation/1 -> PID_C/1, Transfer Fcn/1
  PID Controller/1 -> Saturation/1
  Transfer Fcn/1 -> PID/1
  Ref/1 -> PID Controller/1
